simulink model "Test"  (R2024a)
settings: Solver=VariableStepAuto  StartTime=0.0  StopTime=350  RelTol=1e-3
libraries: eeGeneralControl x2, simulink x1
settings Model: Creator=rocke  LastModifiedBy=rocke

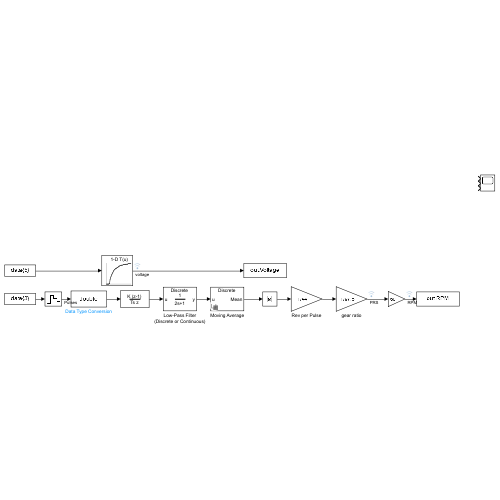
[thumbnail: Simulink's stored preview of the top-level diagram]
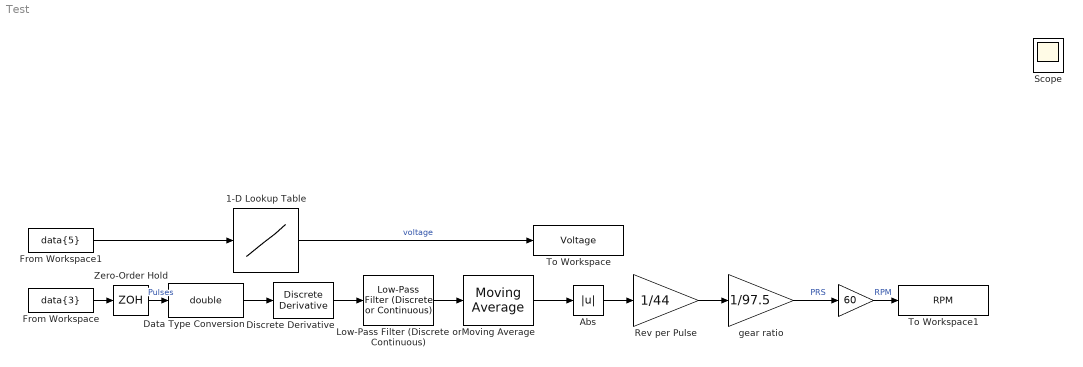
== system Test ==
  " " : Gain  Gain=60
  1-D Lookup Table : Lookup_n-D  NumberOfTableDimensions=1  BreakpointsForDimension1=[0 5 10 15 20 25 30 35 40 45 50 55 60 65 70 75 80 85 90 95 100 105 110 115 120 125 130 135 140 145 150 155 160 165 170 175 180 185 190 195 200 205 210 215 220 225 230 235 240 245 250 255]  Table=[0;0.01;0.029999999999999999;0.050000000000000003;0.10000000000000001;0.13;0.17999999999999999;0.23000000000000001;2.5;3.0800000000000001;3.77;4.54;5.0800000000000001;5.5499999999999998;6.0499999999999998;6.5;6.9699999999999998;7.2300000000000004;7.5099999999999998;7.7199999999999998;7.9000000000000004;8.0899999999999999;8.2799999999999994;8.4000000000000004;8.5600000000000005;8.6500000000000004;8.8699999999999992;9.3000000000000007;9.2699999999999996;9.3300000000000001;9.4499999999999993;9.5099999999999998;9.5899999999999999;9.6600000000000001;9.7400000000000002;9.8200000000000003;9.8900000000000006;9.9100000000000001;9.9600000000000009;10.039999999999999;10.08;10.109999999999999;10.140000000000001;10.199999999999999;10.26;10.31;10.369999999999999;10.43;10.470000000000001;10.470000000000001;10.52;10.74]  InternalRulePriority=Speed  RndMeth=Simplest
  Abs : Abs  SaturateOnIntegerOverflow=off
  Data Type Conversion : DataTypeConversion  OutDataTypeStr=double  SaturateOnIntegerOverflow=off  RndMeth=Floor
  Discrete Derivative : simulink/Discrete/Discrete Derivative  gainval=1.0  ICPrevScaledInput=0.0  OutMin=[]  OutMax=[]  OutDataType=fixdt(1, 16)  OutScaling=2^-10  DoSatur=off
  From Workspace : FromWorkspace  VariableName=data{3}  SampleTime=0.01
  From Workspace1 : FromWorkspace  VariableName=data{5}
  Low-Pass Filter (Discrete or Continuous) : eeGeneralControl/Low-Pass Filter (Discrete or Continuous)  K=1  T=2  B=inf  A=-inf  init_option=Inherited from block input  x0=0  Ts=-1
  Moving Average : eeGeneralControl/Moving Average  VariantControl=Variant1  LabelModeActiveChoice=Discrete  f=1000  x0=0  BufferSize=8192  Ts=-1
      settings: LibrarySourceBlock=ee_sl_lib/General Control/Moving Average
  Rev per Pulse : Gain  Gain=1/44
  Scope : Scope  NumInputPorts=3
  To Workspace : ToWorkspace  VariableName=Voltage  SaveFormat=Timeseries  SampleTime=-1
      settings: Decimation=2
  To Workspace1 : ToWorkspace  VariableName=RPM  SaveFormat=Timeseries  SampleTime=-1
      settings: Decimation=2
  Zero-Order Hold : ZeroOrderHold  SampleTime=-1
  gear ratio : Gain  Gain=1/97.5
  wires:
  From Workspace/1 -> Zero-Order Hold/1
  gear ratio/1 -> " "/1  "PRS"
  Low-Pass Filter (Discrete or Continuous)/1 -> Moving Average/1
  Rev per Pulse/1 -> gear ratio/1
  Discrete Derivative/1 -> Low-Pass Filter (Discrete or Continuous)/1
  Data Type Conversion/1 -> Discrete Derivative/1
  Moving Average/1 -> Abs/1
  Zero-Order Hold/1 -> Data Type Conversion/1  "Pulses"
  " "/1 -> To Workspace1/1  "RPM"
  From Workspace1/1 -> 1-D Lookup Table/1
  1-D Lookup Table/1 -> To Workspace/1  "voltage"
  Abs/1 -> Rev per Pulse/1
